simulink model "qless_forgetting_factor_16x16"  (R2021a)
settings: Solver=FixedStepDiscrete  StartTime=0.0  StopTime=stoptime*inf  RelTol=1e-3
InitFcn:
  | qless_init_16chan_fi
undefined symbols (not defined in the file): fc, numArrayElements, physconst, srcAngles, sv, Ts
libraries: hdlsllib x137, commfilt2 x4, commrfcorlib x3, commsync2 x3, commrflib2 x2, commrandsrc3 x2, phasedtxrxlib x2, commdigbbndcpm2 x1, simulink x1, embreciprocals x1, commdigbbndpm3 x1
(part 4 of 22)

== system qless_forgetting_factor_16x16/MVDR_QLess_HDL/Complex Partial-Systolic Matrix Solve Using Q-less QR Decomposition with Forgetting Factor Manually Tiled n=16/Complex Partial-Systolic Q-less QR with Forgetting Factor/Complex Partial-Systolic Q-less QR with Forgetting Factor Manually tiled/Complex Partial-Systolic Q-less QR Decomposition with Forgetting Factor Section Constant pivot9 ==
  "A(i, :)^T" : Inport
  validIn : Inport  Port=2
  restart : Inport  Port=3
  Complex Partial-Systolic Q-less QR Row Rotations : Subsystem  mask(QR Complex Row Rotations){n=n, pivot=pivot}
      mask prompts: n "fixed:emblib:ColumnsInA"
      mask help: fixed:emblib:ComplexRowRotationsFullDescription
      mask DialogControl n Prompt: Number of columns in matrix A
  Data Type Conversion{,2..6} (6 alike) : DataTypeConversion  OutDataTypeStr=boolean
  Forgetting Factor : Gain  Gain=forgettingFactor  OutDataTypeStr=Inherit: Same as input
  Partial-Systolic Q-less QR with Forgetting Factor Memory Controller : Subsystem  TreatAsAtomicUnit=on  mask(Burst Q-less QR QR Memory Controller){n=n}
      mask prompts: n "fixed:emblib:ColumnsInA"
      mask help: fixed:emblib:MemoryControllerDescription
      mask DialogControl n Prompt: Number of columns in matrix A
  Same Datatype : Subsystem  TreatAsAtomicUnit=on
  Terminator : Terminator
  "R(i, :)^T" : Outport  VectorParamsAs1DForOutWhenUnconnected=off
  validR : Outport  Port=2  VectorParamsAs1DForOutWhenUnconnected=off
  yOut : Outport  Port=3  VectorParamsAs1DForOutWhenUnconnected=off
  validY : Outport  Port=4  VectorParamsAs1DForOutWhenUnconnected=off
  ready : Outport  Port=5  VectorParamsAs1DForOutWhenUnconnected=off
  wires:
  "A(i, :)^T"/1 -> Same Datatype/2(Reference), Partial-Systolic Q-less QR with Forgetting Factor Memory Controller/2(aIn)
  restart/1 -> Data Type Conversion2/1
  Complex Partial-Systolic Q-less QR Row Rotations/3(validOut) -> Data Type Conversion3/1
  Partial-Systolic Q-less QR with Forgetting Factor Memory Controller/4(validOut) -> Data Type Conversion5/1
  validIn/1 -> Data Type Conversion/1
  Partial-Systolic Q-less QR with Forgetting Factor Memory Controller/2(yOut) -> Complex Partial-Systolic Q-less QR Row Rotations/2(y)
  Same Datatype/1(DataOut) -> Partial-Systolic Q-less QR with Forgetting Factor Memory Controller/1(xIn)
  Partial-Systolic Q-less QR with Forgetting Factor Memory Controller/5(ready) -> Data Type Conversion6/1
  Complex Partial-Systolic Q-less QR Row Rotations/2(yOut) -> yOut/1
  Complex Partial-Systolic Q-less QR Row Rotations/4(ready) -> Terminator/1
  Partial-Systolic Q-less QR with Forgetting Factor Memory Controller/3(process) -> Data Type Conversion4/1
  Complex Partial-Systolic Q-less QR Row Rotations/1(xOut) -> Forgetting Factor/1
  Partial-Systolic Q-less QR with Forgetting Factor Memory Controller/1(xOut) -> Complex Partial-Systolic Q-less QR Row Rotations/1(x), "R(i, :)^T"/1
  Forgetting Factor/1 -> Same Datatype/1(Data)
  Data Type Conversion/1 -> Partial-Systolic Q-less QR with Forgetting Factor Memory Controller/3(validIn)
  Data Type Conversion2/1 -> Complex Partial-Systolic Q-less QR Row Rotations/4(restart), Partial-Systolic Q-less QR with Forgetting Factor Memory Controller/5(restart)
  Data Type Conversion3/1 -> Partial-Systolic Q-less QR with Forgetting Factor Memory Controller/4(validElim), validY/1
  Data Type Conversion5/1 -> validR/1
  Data Type Conversion6/1 -> ready/1
  Data Type Conversion4/1 -> Complex Partial-Systolic Q-less QR Row Rotations/3(validIn)

== system qless_forgetting_factor_16x16/MVDR_QLess_HDL/Complex Partial-Systolic Matrix Solve Using Q-less QR Decomposition with Forgetting Factor Manually Tiled n=16/Complex Partial-Systolic Q-less QR with Forgetting Factor/Complex Partial-Systolic Q-less QR with Forgetting Factor Manually tiled/Lengthen ==
  u : Inport
  Lengthen : MATLAB Function  TreatAsAtomicUnit=on
  y : Outport
  wires:
  Lengthen/1(y) -> y/1
  u/1 -> Lengthen/1(u)

== system qless_forgetting_factor_16x16/MVDR_QLess_HDL/Complex Partial-Systolic Matrix Solve Using Q-less QR Decomposition with Forgetting Factor Manually Tiled n=16/Complex Partial-Systolic Q-less QR with Forgetting Factor/Complex Partial-Systolic Q-less QR with Forgetting Factor Manually tiled/Lengthen1 ==
  u : Inport
  Lengthen : MATLAB Function  TreatAsAtomicUnit=on
  y : Outport
  wires:
  Lengthen/1(y) -> y/1
  u/1 -> Lengthen/1(u)

== system qless_forgetting_factor_16x16/MVDR_QLess_HDL/Complex Partial-Systolic Matrix Solve Using Q-less QR Decomposition with Forgetting Factor Manually Tiled n=16/Complex Partial-Systolic Q-less QR with Forgetting Factor/Complex Partial-Systolic Q-less QR with Forgetting Factor Manually tiled/Lengthen10 ==
  u : Inport
  Lengthen : MATLAB Function  TreatAsAtomicUnit=on
  y : Outport
  wires:
  Lengthen/1(y) -> y/1
  u/1 -> Lengthen/1(u)

== system qless_forgetting_factor_16x16/MVDR_QLess_HDL/Complex Partial-Systolic Matrix Solve Using Q-less QR Decomposition with Forgetting Factor Manually Tiled n=16/Complex Partial-Systolic Q-less QR with Forgetting Factor/Complex Partial-Systolic Q-less QR with Forgetting Factor Manually tiled/Lengthen11 ==
  u : Inport
  Lengthen : MATLAB Function  TreatAsAtomicUnit=on
  y : Outport
  wires:
  Lengthen/1(y) -> y/1
  u/1 -> Lengthen/1(u)

== system qless_forgetting_factor_16x16/MVDR_QLess_HDL/Complex Partial-Systolic Matrix Solve Using Q-less QR Decomposition with Forgetting Factor Manually Tiled n=16/Complex Partial-Systolic Q-less QR with Forgetting Factor/Complex Partial-Systolic Q-less QR with Forgetting Factor Manually tiled/Lengthen12 ==
  u : Inport
  Lengthen : MATLAB Function  TreatAsAtomicUnit=on
  y : Outport
  wires:
  Lengthen/1(y) -> y/1
  u/1 -> Lengthen/1(u)

== system qless_forgetting_factor_16x16/MVDR_QLess_HDL/Complex Partial-Systolic Matrix Solve Using Q-less QR Decomposition with Forgetting Factor Manually Tiled n=16/Complex Partial-Systolic Q-less QR with Forgetting Factor/Complex Partial-Systolic Q-less QR with Forgetting Factor Manually tiled/Lengthen13 ==
  u : Inport
  Lengthen : MATLAB Function  TreatAsAtomicUnit=on
  y : Outport
  wires:
  Lengthen/1(y) -> y/1
  u/1 -> Lengthen/1(u)

== system qless_forgetting_factor_16x16/MVDR_QLess_HDL/Complex Partial-Systolic Matrix Solve Using Q-less QR Decomposition with Forgetting Factor Manually Tiled n=16/Complex Partial-Systolic Q-less QR with Forgetting Factor/Complex Partial-Systolic Q-less QR with Forgetting Factor Manually tiled/Lengthen14 ==
  u : Inport
  Lengthen : MATLAB Function  TreatAsAtomicUnit=on
  y : Outport
  wires:
  Lengthen/1(y) -> y/1
  u/1 -> Lengthen/1(u)

== system qless_forgetting_factor_16x16/MVDR_QLess_HDL/Complex Partial-Systolic Matrix Solve Using Q-less QR Decomposition with Forgetting Factor Manually Tiled n=16/Complex Partial-Systolic Q-less QR with Forgetting Factor/Complex Partial-Systolic Q-less QR with Forgetting Factor Manually tiled/Lengthen2 ==
  u : Inport
  Lengthen : MATLAB Function  TreatAsAtomicUnit=on
  y : Outport
  wires:
  Lengthen/1(y) -> y/1
  u/1 -> Lengthen/1(u)

== system qless_forgetting_factor_16x16/MVDR_QLess_HDL/Complex Partial-Systolic Matrix Solve Using Q-less QR Decomposition with Forgetting Factor Manually Tiled n=16/Complex Partial-Systolic Q-less QR with Forgetting Factor/Complex Partial-Systolic Q-less QR with Forgetting Factor Manually tiled/Lengthen3 ==
  u : Inport
  Lengthen : MATLAB Function  TreatAsAtomicUnit=on
  y : Outport
  wires:
  Lengthen/1(y) -> y/1
  u/1 -> Lengthen/1(u)

== system qless_forgetting_factor_16x16/MVDR_QLess_HDL/Complex Partial-Systolic Matrix Solve Using Q-less QR Decomposition with Forgetting Factor Manually Tiled n=16/Complex Partial-Systolic Q-less QR with Forgetting Factor/Complex Partial-Systolic Q-less QR with Forgetting Factor Manually tiled/Lengthen4 ==
  u : Inport
  Lengthen : MATLAB Function  TreatAsAtomicUnit=on
  y : Outport
  wires:
  Lengthen/1(y) -> y/1
  u/1 -> Lengthen/1(u)

== system qless_forgetting_factor_16x16/MVDR_QLess_HDL/Complex Partial-Systolic Matrix Solve Using Q-less QR Decomposition with Forgetting Factor Manually Tiled n=16/Complex Partial-Systolic Q-less QR with Forgetting Factor/Complex Partial-Systolic Q-less QR with Forgetting Factor Manually tiled/Lengthen5 ==
  u : Inport
  Lengthen : MATLAB Function  TreatAsAtomicUnit=on
  y : Outport
  wires:
  Lengthen/1(y) -> y/1
  u/1 -> Lengthen/1(u)

== system qless_forgetting_factor_16x16/MVDR_QLess_HDL/Complex Partial-Systolic Matrix Solve Using Q-less QR Decomposition with Forgetting Factor Manually Tiled n=16/Complex Partial-Systolic Q-less QR with Forgetting Factor/Complex Partial-Systolic Q-less QR with Forgetting Factor Manually tiled/Lengthen6 ==
  u : Inport
  Lengthen : MATLAB Function  TreatAsAtomicUnit=on
  y : Outport
  wires:
  Lengthen/1(y) -> y/1
  u/1 -> Lengthen/1(u)

== system qless_forgetting_factor_16x16/MVDR_QLess_HDL/Complex Partial-Systolic Matrix Solve Using Q-less QR Decomposition with Forgetting Factor Manually Tiled n=16/Complex Partial-Systolic Q-less QR with Forgetting Factor/Complex Partial-Systolic Q-less QR with Forgetting Factor Manually tiled/Lengthen7 ==
  u : Inport
  Lengthen : MATLAB Function  TreatAsAtomicUnit=on
  y : Outport
  wires:
  Lengthen/1(y) -> y/1
  u/1 -> Lengthen/1(u)

== system qless_forgetting_factor_16x16/MVDR_QLess_HDL/Complex Partial-Systolic Matrix Solve Using Q-less QR Decomposition with Forgetting Factor Manually Tiled n=16/Complex Partial-Systolic Q-less QR with Forgetting Factor/Complex Partial-Systolic Q-less QR with Forgetting Factor Manually tiled/Lengthen8 ==
  u : Inport
  Lengthen : MATLAB Function  TreatAsAtomicUnit=on
  y : Outport
  wires:
  Lengthen/1(y) -> y/1
  u/1 -> Lengthen/1(u)

== system qless_forgetting_factor_16x16/MVDR_QLess_HDL/Complex Partial-Systolic Matrix Solve Using Q-less QR Decomposition with Forgetting Factor Manually Tiled n=16/Complex Partial-Systolic Q-less QR with Forgetting Factor/Complex Partial-Systolic Q-less QR with Forgetting Factor Manually tiled/Lengthen9 ==
  u : Inport
  Lengthen : MATLAB Function  TreatAsAtomicUnit=on
  y : Outport
  wires:
  Lengthen/1(y) -> y/1
  u/1 -> Lengthen/1(u)

== system qless_forgetting_factor_16x16/MVDR_QLess_HDL/Complex Partial-Systolic Matrix Solve Using Q-less QR Decomposition with Forgetting Factor Manually Tiled n=16/Complex Partial-Systolic Q-less QR with Forgetting Factor/Partial-Systolic Q-less QR with Forgetting Factor Output Memory Manager/Partial-Systolic Q-less QR Output Memory Manager1 ==
  RtransposeIn : Inport
  validIn : Inport  Port=2
  restart : Inport  Port=3
  Delay3 : Delay  DelayLength=1
  Delay5 : Delay  DelayLength=1
  Partial-Systolic Q-less QR Output State Machine : MATLAB Function  TreatAsAtomicUnit=on  mask{m=m, n=n}
      mask prompts: m "fixed:emblib:RowsInA"; n "fixed:emblib:ColumnsInA"
  Save Matrix Row : Subsystem  mask{n=n}
      mask prompts: n "Number of elements in vactor dataIn"
      mask help: The n-by-n input matrix is flattened to an1-by-n^2 row. The row selector is a 1-by-n vector of logical values with a true element corresponding to a row of the matrix to save. There is one cycle delay between input and output.
      mask Display: disp('Save matrix row')
  RtransposeOut : Outport
  validOut : Outport  Port=2
  wires:
  Save Matrix Row/1(matrixOut) -> RtransposeOut/1
  Partial-Systolic Q-less QR Output State Machine/2(validOut) -> Delay3/1
  restart/1 -> Partial-Systolic Q-less QR Output State Machine/2(restart)
  Partial-Systolic Q-less QR Output State Machine/1(writeEnable) -> Save Matrix Row/2(rowSelector)
  Delay5/1 -> Save Matrix Row/1(matrixIn)
  Delay3/1 -> validOut/1
  RtransposeIn/1 -> Delay5/1
  validIn/1 -> Partial-Systolic Q-less QR Output State Machine/1(validIn)

== system qless_forgetting_factor_16x16/MVDR_QLess_HDL/Complex Partial-Systolic Matrix Solve Using Q-less QR Decomposition with Forgetting Factor Manually Tiled n=16/Complex Q-less QR Forward Backward Substitute/Complex Burst Back Substitute with Matrix Output1/Back substitute logic ==
  inverseElement : Inport
  inverseShift : Inport  Port=2
  rIn : Inport  Port=3
  cIn : Inport  Port=4
  validIn : Inport  Port=5
  start : Inport  Port=6
  restart : Inport  Port=7
  Add products : Sum  OutDataTypeStr=Inherit: Same as first input
  Back substitute state machine : MATLAB Function  TreatAsAtomicUnit=on
  Complex-Complex Multiply : Subsystem  TreatAsAtomicUnit=on
  Complex-Real Multiply : Subsystem  TreatAsAtomicUnit=on
  Delay{3..4,8,11} (4 alike) : Delay  DelayLength=1
  Same Datatype : Subsystem  TreatAsAtomicUnit=on
  Same Datatype1 : Subsystem  TreatAsAtomicUnit=on
  Same Datatype2 : Subsystem  TreatAsAtomicUnit=on
  Same Datatype3 : Subsystem  TreatAsAtomicUnit=on
  Subtract sumOfProducts from qtbRow : Sum  Inputs=+-  OutDataTypeStr=Inherit: Same as first input
  Variable shift : Subsystem  TreatAsAtomicUnit=on
  X : Outport  VectorParamsAs1DForOutWhenUnconnected=off
  validOut : Outport  Port=2  VectorParamsAs1DForOutWhenUnconnected=off
  rowReady : Outport  Port=3  VectorParamsAs1DForOutWhenUnconnected=off
  ready : Outport  Port=4  VectorParamsAs1DForOutWhenUnconnected=off
  wires:
  Back substitute state machine/10(xMatrix) -> X/1
  Delay3/1 -> Same Datatype3/1(Data)
  Same Datatype3/1(DataOut) -> Back substitute state machine/11(finalMultipliedRow)
  Delay4/1 -> Same Datatype2/1(Data)
  Same Datatype2/1(DataOut) -> Back substitute state machine/10(multipliedRow)
  Delay8/1 -> Same Datatype1/1(Data)
  Same Datatype1/1(DataOut) -> Back substitute state machine/9(addedRow)
  Delay11/1 -> Same Datatype/1(Data)
  Same Datatype/1(DataOut) -> Back substitute state machine/8(subtractedRow)
  Back substitute state machine/3(rowToAdd1) -> Add products/1
  Back substitute state machine/4(rowToAdd2) -> Add products/2
  Back substitute state machine/6(rElement) -> Complex-Complex Multiply/2(multiplier)
  Back substitute state machine/5(rowToMultiply) -> Complex-Complex Multiply/1(row)
  inverseElement/1 -> Back substitute state machine/1(inverseElement)
  rIn/1 -> Back substitute state machine/3(rIn)
  cIn/1 -> Same Datatype3/2(Reference), Same Datatype2/2(Reference), Same Datatype1/2(Reference), Same Datatype/2(Reference), Back substitute state machine/4(cIn)
  validIn/1 -> Back substitute state machine/5(validIn)
  start/1 -> Back substitute state machine/6(start)
  restart/1 -> Back substitute state machine/7(restart)
  Back substitute state machine/11(ready) -> ready/1
  Back substitute state machine/12(rowReady) -> rowReady/1
  Back substitute state machine/9(shiftValue) -> Variable shift/2(shiftValue)
  inverseShift/1 -> Back substitute state machine/2(inverseShift)
  Back substitute state machine/13(validOut) -> validOut/1
  Back substitute state machine/8(reciprocal) -> Complex-Real Multiply/2(multiplier)
  Back substitute state machine/7(finalRowToMultiply) -> Complex-Real Multiply/1(row)
  Complex-Real Multiply/1(output) -> Variable shift/1(x)
  Variable shift/1(y) -> Delay3/1
  Complex-Complex Multiply/1(output) -> Delay4/1
  Back substitute state machine/2(rowToSubtract2) -> Subtract sumOfProducts from qtbRow/2
  Back substitute state machine/1(rowToSubtract1) -> Subtract sumOfProducts from qtbRow/1
  Subtract sumOfProducts from qtbRow/1 -> Delay11/1
  Add products/1 -> Delay8/1

== system qless_forgetting_factor_16x16/MVDR_QLess_HDL/Complex Partial-Systolic Matrix Solve Using Q-less QR Decomposition with Forgetting Factor Manually Tiled n=16/Complex Q-less QR Forward Backward Substitute/Complex Burst Back Substitute with Matrix Output1/Reciprocal of the diagonal element ==
  rIn : Inport
  start : Inport  Port=2
  validIn : Inport  Port=3
  Positive Normalized Reciprocal HDL Optimized : Subsystem  mask(Positive Normalized Reciprocal HDL Optimized){}
      mask help: fixed:emblib:PositiveNormalizedReciprocalFullDescription
      mask Help: For internal use only. This feature is intentionally undocumented. Its behavior may change, or it may be removed in a future release.
      mask Display:
      | text(0.5,0.7,'u > 0','texmode','on','HorizontalAlignment','center')
      | text(0.5,0.5,'2^e y = 1/u','texmode','on','HorizontalAlignment','center')
      | text(0.5,0.3,'0.5 < y \leq 1','texmode','on','HorizontalAlignment','center')
  Select diagonal element : MATLAB Function  TreatAsAtomicUnit=on
  inverseElement : Outport  VectorParamsAs1DForOutWhenUnconnected=off
  inverseShift : Outport  Port=2  VectorParamsAs1DForOutWhenUnconnected=off
  validOut : Outport  Port=3  VectorParamsAs1DForOutWhenUnconnected=off
  wires:
  Positive Normalized Reciprocal HDL Optimized/2(e) -> inverseShift/1
  Positive Normalized Reciprocal HDL Optimized/3(validOut) -> validOut/1
  Select diagonal element/1(y) -> Positive Normalized Reciprocal HDL Optimized/1(u)
  rIn/1 -> Select diagonal element/1(rIn)
  Select diagonal element/2(validOut) -> Positive Normalized Reciprocal HDL Optimized/2(validIn)
  start/1 -> Select diagonal element/2(start)
  validIn/1 -> Select diagonal element/3(validIn)
  Positive Normalized Reciprocal HDL Optimized/1(y) -> inverseElement/1

== system qless_forgetting_factor_16x16/MVDR_QLess_HDL/Complex Partial-Systolic Matrix Solve Using Q-less QR Decomposition with Forgetting Factor Manually Tiled n=16/Complex Q-less QR Forward Backward Substitute/Complex Burst Forward Substitute with Matrix Output/Forward substitute logic ==
  inverseElement : Inport
  inverseShift : Inport  Port=2
  rIn : Inport  Port=3
  cIn : Inport  Port=4
  validIn : Inport  Port=5
  start : Inport  Port=6
  restart : Inport  Port=7
  Add products : Sum  OutDataTypeStr=Inherit: Same as first input
  Complex-Complex Multiply1 : Subsystem  TreatAsAtomicUnit=on
  Complex-Real Multiply : Subsystem  TreatAsAtomicUnit=on
  Delay{3..4,8,11} (4 alike) : Delay  DelayLength=1
  Forward substitute state machine : MATLAB Function  TreatAsAtomicUnit=on
  Same Datatype : Subsystem  TreatAsAtomicUnit=on
  Same Datatype1 : Subsystem  TreatAsAtomicUnit=on
  Same Datatype2 : Subsystem  TreatAsAtomicUnit=on
  Same Datatype3 : Subsystem  TreatAsAtomicUnit=on
  Subtract sumOfProducts from qtbRow : Sum  Inputs=+-  OutDataTypeStr=Inherit: Same as first input
  Variable shift : Subsystem  TreatAsAtomicUnit=on
  X : Outport  VectorParamsAs1DForOutWhenUnconnected=off
  validOut : Outport  Port=2  VectorParamsAs1DForOutWhenUnconnected=off
  rowReady : Outport  Port=3  VectorParamsAs1DForOutWhenUnconnected=off
  ready : Outport  Port=4  VectorParamsAs1DForOutWhenUnconnected=off
  wires:
  Forward substitute state machine/10(xMatrix) -> X/1
  Forward substitute state machine/13(validOut) -> validOut/1
  Delay3/1 -> Same Datatype3/1(Data)
  Same Datatype3/1(DataOut) -> Forward substitute state machine/11(finalMultipliedRow)
  Delay4/1 -> Same Datatype2/1(Data)
  Same Datatype2/1(DataOut) -> Forward substitute state machine/10(multipliedRow)
  Delay8/1 -> Same Datatype1/1(Data)
  Same Datatype1/1(DataOut) -> Forward substitute state machine/9(addedRow)
  Delay11/1 -> Same Datatype/1(Data)
  Same Datatype/1(DataOut) -> Forward substitute state machine/8(subtractedRow)
  Forward substitute state machine/3(rowToAdd1) -> Add products/1
  Forward substitute state machine/4(rowToAdd2) -> Add products/2
  Forward substitute state machine/6(rElement) -> Complex-Complex Multiply1/2(multiplier)
  Forward substitute state machine/5(rowToMultiply) -> Complex-Complex Multiply1/1(row)
  inverseElement/1 -> Forward substitute state machine/1(inverseElement)
  rIn/1 -> Forward substitute state machine/3(rIn)
  cIn/1 -> Same Datatype3/2(Reference), Same Datatype2/2(Reference), Same Datatype1/2(Reference), Same Datatype/2(Reference), Forward substitute state machine/4(cIn)
  validIn/1 -> Forward substitute state machine/5(validIn)
  start/1 -> Forward substitute state machine/6(start)
  restart/1 -> Forward substitute state machine/7(restart)
  Forward substitute state machine/11(ready) -> ready/1
  Forward substitute state machine/12(rowReady) -> rowReady/1
  Forward substitute state machine/9(shiftValue) -> Variable shift/2(shiftValue)
  inverseShift/1 -> Forward substitute state machine/2(inverseShift)
  Forward substitute state machine/8(reciprocal) -> Complex-Real Multiply/2(multiplier)
  Forward substitute state machine/7(finalRowToMultiply) -> Complex-Real Multiply/1(row)
  Complex-Real Multiply/1(output) -> Variable shift/1(x)
  Variable shift/1(y) -> Delay3/1
  Complex-Complex Multiply1/1(output) -> Delay4/1
  Forward substitute state machine/2(rowToSubtract2) -> Subtract sumOfProducts from qtbRow/2
  Forward substitute state machine/1(rowToSubtract1) -> Subtract sumOfProducts from qtbRow/1
  Subtract sumOfProducts from qtbRow/1 -> Delay11/1
  Add products/1 -> Delay8/1

== system qless_forgetting_factor_16x16/MVDR_QLess_HDL/Complex Partial-Systolic Matrix Solve Using Q-less QR Decomposition with Forgetting Factor Manually Tiled n=16/Complex Q-less QR Forward Backward Substitute/Complex Burst Forward Substitute with Matrix Output/Reciprocal of the diagonal element ==
  rIn : Inport
  start : Inport  Port=2
  validIn : Inport  Port=3
  Positive Normalized Reciprocal HDL Optimized : Subsystem  mask(Positive Normalized Reciprocal HDL Optimized){}
      mask help: fixed:emblib:PositiveNormalizedReciprocalFullDescription
      mask Help: For internal use only. This feature is intentionally undocumented. Its behavior may change, or it may be removed in a future release.
      mask Display:
      | text(0.5,0.7,'u > 0','texmode','on','HorizontalAlignment','center')
      | text(0.5,0.5,'2^e y = 1/u','texmode','on','HorizontalAlignment','center')
      | text(0.5,0.3,'0.5 < y \leq 1','texmode','on','HorizontalAlignment','center')
  Select diagonal element : MATLAB Function  TreatAsAtomicUnit=on
  inverseElement : Outport  VectorParamsAs1DForOutWhenUnconnected=off
  inverseShift : Outport  Port=2  VectorParamsAs1DForOutWhenUnconnected=off
  validOut : Outport  Port=3  VectorParamsAs1DForOutWhenUnconnected=off
  wires:
  Positive Normalized Reciprocal HDL Optimized/2(e) -> inverseShift/1
  Positive Normalized Reciprocal HDL Optimized/3(validOut) -> validOut/1
  Select diagonal element/1(y) -> Positive Normalized Reciprocal HDL Optimized/1(u)
  rIn/1 -> Select diagonal element/1(rIn)
  Select diagonal element/2(validOut) -> Positive Normalized Reciprocal HDL Optimized/2(validIn)
  start/1 -> Select diagonal element/2(start)
  validIn/1 -> Select diagonal element/3(validIn)
  Positive Normalized Reciprocal HDL Optimized/1(y) -> inverseElement/1

== system qless_forgetting_factor_16x16/MVDR_QLess_HDL/Complex Partial-Systolic Matrix Solve Using Q-less QR Decomposition with Forgetting Factor Manually Tiled n=16/Complex Q-less QR Forward Backward Substitute/Partial-Systolic Matrix Solve Q-less QR B Buffer Manager/Save Matrix B ==
  matrixIn : Inport  Partition=on  PartitionDimension=1  PartitionWidth=n  PartitionOffset=0
  validIn : Inport  Port=2
  restart : Inport  Port=3
  Enabled Delay : MATLAB Function  TreatAsAtomicUnit=on
  For Each : ForEach  DisableCoverage=on
  Reshape : Reshape  OutputDimensionality=Column vector (2-D)
  matrixOut : Outport  ConcatenationDimension=1
  wires:
  restart/1 -> Enabled Delay/3(restart)
  validIn/1 -> Enabled Delay/2(writeEnable)
  matrixIn/1 -> Enabled Delay/1(dataIn)
  Enabled Delay/1(dataOut) -> Reshape/1
  Reshape/1 -> matrixOut/1

== system qless_forgetting_factor_16x16/MVDR_QLess_HDL/Complex Partial-Systolic Matrix Solve Using Q-less QR Decomposition with Forgetting Factor Manually Tiled n=16/Complex Q-less QR Forward Backward Substitute/Partial-Systolic Matrix Solve Q-less QR Forward Substitute Memory Manager/Save Matrix B ==
  matrixIn : Inport  Partition=on  PartitionDimension=1  PartitionWidth=n  PartitionOffset=0
  validIn : Inport  Port=2
  restart : Inport  Port=3
  Enabled Delay : MATLAB Function  TreatAsAtomicUnit=on
  For Each : ForEach  DisableCoverage=on
  Reshape : Reshape  OutputDimensionality=Column vector (2-D)
  matrixOut : Outport  ConcatenationDimension=1
  wires:
  restart/1 -> Enabled Delay/3(restart)
  validIn/1 -> Enabled Delay/2(writeEnable)
  matrixIn/1 -> Enabled Delay/1(dataIn)
  Enabled Delay/1(dataOut) -> Reshape/1
  Reshape/1 -> matrixOut/1

== system qless_forgetting_factor_16x16/MVDR_QLess_HDL/Complex Partial-Systolic Matrix Solve Using Q-less QR Decomposition with Forgetting Factor Manually Tiled n=16/Complex Q-less QR Forward Backward Substitute/Partial-Systolic Matrix Solve Q-less QR Output Manager/Save Matrix ==
  matrixIn : Inport  Partition=on  PartitionDimension=1  PartitionWidth=n  PartitionOffset=0
  validIn : Inport  Port=2
  restart : Inport  Port=3
  Enabled Delay : MATLAB Function  TreatAsAtomicUnit=on
  For Each : ForEach  DisableCoverage=on
  Reshape : Reshape  OutputDimensionality=Column vector (2-D)
  matrixOut : Outport  ConcatenationDimension=1
  wires:
  restart/1 -> Enabled Delay/3(restart)
  validIn/1 -> Enabled Delay/2(writeEnable)
  matrixIn/1 -> Enabled Delay/1(dataIn)
  Enabled Delay/1(dataOut) -> Reshape/1
  Reshape/1 -> matrixOut/1

== system qless_forgetting_factor_16x16/MVDR_QLess_HDL/Normalize Response/MVDR Weight Update/Inner Product/Element-wise complex product ==
  u : Inport  Partition=on  PartitionDimension=1  PartitionWidth=1  PartitionOffset=0
  v : Inport  Port=2  Partition=on  PartitionDimension=1  PartitionWidth=1  PartitionOffset=0
  For Each : ForEach  DisableCoverage=on
  HDL Complex Multiply : Subsystem  mask(HDL Complex Multiplier (3 Multiply, 5 Add)){D1=2, D2=1, D3=1, D4=1, D5=1}
      mask help:
      | Xilinx devices:
      | - Set D1 = 1 or 2 to trade off speed & FF resources
      | - Set D2-D5 = 1 to fully leverage DSP48 pipelines
      | - Use sync reset
      |
      | Intel FPGAs:
      | - Set D1 = 1 or 2 depending on device family
      | - Set D5 = 1; D2, D3, D4 = 0
      | - Use async reset
      mask init:
      | delay = D1+D2+D3+D4+D5;
      mask Display:
      | fprintf('Delay=%d',delay);
      | port_label('input',1,'z1');
      | port_label('input',2,'z2');
  y : Outport  ConcatenationDimension=1
  wires:
  v/1 -> HDL Complex Multiply/2(In2)
  HDL Complex Multiply/1(Out1) -> y/1
  u/1 -> HDL Complex Multiply/1(In1)

== system qless_forgetting_factor_16x16/MVDR_QLess_HDL/Normalize Response/MVDR Weight Update/Inner Product/Tree Sum with Distributed Pipelining ==
  In1 : Inport
  Delay3 : Delay  DelayLength=ceil(log2(numArrayElements))
  Tree Sum of Elements : Sum  Inputs=+
  Out1 : Outport
  wires:
  Delay3/1 -> Out1/1
  In1/1 -> Tree Sum of Elements/1
  Tree Sum of Elements/1 -> Delay3/1

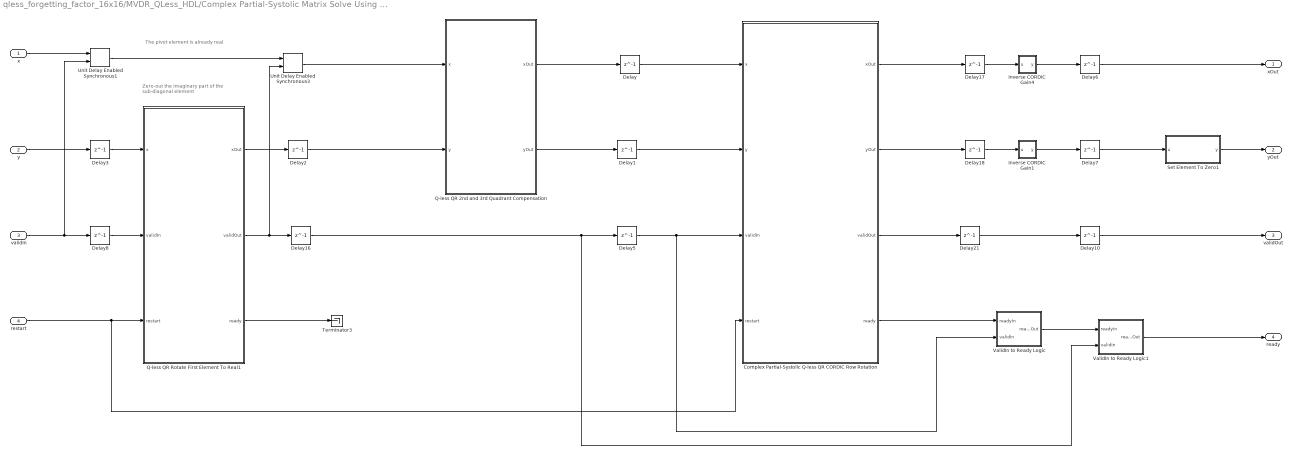
== system qless_forgetting_factor_16x16/MVDR_QLess_HDL/Complex Partial-Systolic Matrix Solve Using Q-less QR Decomposition with Forgetting Factor Manually Tiled n=16/Complex Partial-Systolic Q-less QR with Forgetting Factor/Complex Partial-Systolic Q-less QR with Forgetting Factor Manually tiled/Complex Partial-Systolic Q-less QR Decomposition with Forgetting Factor Section Constant pivot1/Complex Partial-Systolic Q-less QR Row Rotations ==
  note: The pivot element is already real
  note: Zero-out the imaginary part
      | of the sub-diagonal element
  x : Inport
  y : Inport  Port=2
  validIn : Inport  Port=3
  restart : Inport  Port=4
  Complex Partial-Systolic Q-less QR CORDIC Row Rotation : Subsystem  TreatAsAtomicUnit=on  mask(Real Indexed CORDIC Row Rotation){n=n, pivot=pivot}
      mask prompts: n "fixed:emblib:ColumnsInA"
      mask help: fixed:emblib:RealIdxCORDIC
      mask DialogControl n Prompt: Number of columns in matrix A
  Delay{,1..3,5..8,10,16..18,21} (13 alike) : Delay  DelayLength=1
  Inverse CORDIC Gain1 : Subsystem  mask(Inverse CORDIC Gain){}
      mask help: fixed:emblib:InverseCORDICGainDescription
      mask Display: disp('1/An')
  Inverse CORDIC Gain4 : Subsystem  mask(Inverse CORDIC Gain){}
      mask help: fixed:emblib:InverseCORDICGainDescription
      mask Display: disp('1/An')
  Q-less QR 2nd and 3rd Quadrant Compensation : MATLAB Function  TreatAsAtomicUnit=on
  Q-less QR Rotate First Element To Real1 : Subsystem  TreatAsAtomicUnit=on  mask(Rotate First Element To Real){n=n, pivot=pivot}
      mask prompts: n "fixed:emblib:ColumnsInA"
      mask help: fixed:emblib:RotateFirstElementToRealDescription
      mask DialogControl n Prompt: Number of columns in matrix A
  Set Element To Zero1 : Subsystem  mask(Set Element To Zero){n=n, pivot=pivot}
      mask prompts: n "fixed:emblib:ColumnsInA"
      mask help: fixed:emblib:SetElementToZeroDescription
      mask DialogControl n Prompt: Number of columns in matrix A
  Terminator3 : Terminator
  Unit Delay Enabled Synchronous1 : hdlsllib/Discrete/Unit Delay Enabled Synchronous  InitialCondition=0.0  SampleTime=-1
      settings: SourceProductBaseCode=SL
  Unit Delay Enabled Synchronous3 : hdlsllib/Discrete/Unit Delay Enabled Synchronous  InitialCondition=0.0  SampleTime=-1
      settings: SourceProductBaseCode=SL
  ValidIn to Ready Logic : Subsystem
  ValidIn to Ready Logic1 : Subsystem
  xOut : Outport  VectorParamsAs1DForOutWhenUnconnected=off
  yOut : Outport  Port=2  VectorParamsAs1DForOutWhenUnconnected=off
  validOut : Outport  Port=3  VectorParamsAs1DForOutWhenUnconnected=off
  ready : Outport  Port=4  VectorParamsAs1DForOutWhenUnconnected=off
  wires:
  Delay6/1 -> xOut/1
  Complex Partial-Systolic Q-less QR CORDIC Row Rotation/1(xOut) -> Delay17/1
  Q-less QR 2nd and 3rd Quadrant Compensation/1(xOut) -> Delay/1
  Q-less QR 2nd and 3rd Quadrant Compensation/2(yOut) -> Delay1/1
  Delay/1 -> Complex Partial-Systolic Q-less QR CORDIC Row Rotation/1(x)
  Q-less QR Rotate First Element To Real1/2(validOut) -> Unit Delay Enabled Synchronous3/2, Delay16/1
  Q-less QR Rotate First Element To Real1/1(xOut) -> Delay2/1
  Delay1/1 -> Complex Partial-Systolic Q-less QR CORDIC Row Rotation/2(y)
  restart/1 -> Q-less QR Rotate First Element To Real1/3(restart), Complex Partial-Systolic Q-less QR CORDIC Row Rotation/4(restart)
  Delay5/1 -> ValidIn to Ready Logic/2(validIn), Complex Partial-Systolic Q-less QR CORDIC Row Rotation/3(validIn)
  Complex Partial-Systolic Q-less QR CORDIC Row Rotation/4(ready) -> ValidIn to Ready Logic/1(readyIn)
  Complex Partial-Systolic Q-less QR CORDIC Row Rotation/3(validOut) -> Delay21/1
  Complex Partial-Systolic Q-less QR CORDIC Row Rotation/2(yOut) -> Delay18/1
  y/1 -> Delay3/1
  Delay10/1 -> validOut/1
  ValidIn to Ready Logic/1(readyOut) -> ValidIn to Ready Logic1/1(readyIn)
  Delay7/1 -> Set Element To Zero1/1(u)
  Q-less QR Rotate First Element To Real1/3(ready) -> Terminator3/1
  ValidIn to Ready Logic1/1(readyOut) -> ready/1
  Delay21/1 -> Delay10/1
  Delay18/1 -> Inverse CORDIC Gain1/1(u)
  Delay17/1 -> Inverse CORDIC Gain4/1(u)
  Inverse CORDIC Gain4/1(y) -> Delay6/1
  Inverse CORDIC Gain1/1(y) -> Delay7/1
  validIn/1 -> Unit Delay Enabled Synchronous1/2, Delay8/1
  Delay16/1 -> ValidIn to Ready Logic1/2(validIn), Delay5/1
  Delay2/1 -> Q-less QR 2nd and 3rd Quadrant Compensation/2(y)
  Unit Delay Enabled Synchronous3/1 -> Q-less QR 2nd and 3rd Quadrant Compensation/1(x)
  Unit Delay Enabled Synchronous1/1 -> Unit Delay Enabled Synchronous3/1
  x/1 -> Unit Delay Enabled Synchronous1/1
  Delay3/1 -> Q-less QR Rotate First Element To Real1/1(x)
  Delay8/1 -> Q-less QR Rotate First Element To Real1/2(validIn)
  Set Element To Zero1/1(y) -> yOut/1

== system qless_forgetting_factor_16x16/MVDR_QLess_HDL/Complex Partial-Systolic Matrix Solve Using Q-less QR Decomposition with Forgetting Factor Manually Tiled n=16/Complex Partial-Systolic Q-less QR with Forgetting Factor/Complex Partial-Systolic Q-less QR with Forgetting Factor Manually tiled/Complex Partial-Systolic Q-less QR Decomposition with Forgetting Factor Section Constant pivot1/Partial-Systolic Q-less QR with Forgetting Factor Memory Controller ==
  xIn : Inport
  aIn : Inport  Port=2
  validIn : Inport  Port=3
  validElim : Inport  Port=4
  restart : Inport  Port=5
  Delay{,2..4,6} (5 alike) : Delay  DelayLength=1
  MATLAB Function : MATLAB Function  TreatAsAtomicUnit=on
  xOut : Outport  VectorParamsAs1DForOutWhenUnconnected=off
  yOut : Outport  Port=2  VectorParamsAs1DForOutWhenUnconnected=off
  process : Outport  Port=3  VectorParamsAs1DForOutWhenUnconnected=off
  validOut : Outport  Port=4  VectorParamsAs1DForOutWhenUnconnected=off
  ready : Outport  Port=5  VectorParamsAs1DForOutWhenUnconnected=off
  wires:
  Delay/1 -> MATLAB Function/1(xIn)
  Delay2/1 -> MATLAB Function/2(aIn)
  Delay3/1 -> MATLAB Function/3(validIn)
  Delay4/1 -> MATLAB Function/4(validRowRotationInput)
  Delay6/1 -> MATLAB Function/5(restart)
  xIn/1 -> Delay/1  "A"
  aIn/1 -> Delay2/1
  validIn/1 -> Delay3/1  "validIn"
  validElim/1 -> Delay4/1  "validElim"
  restart/1 -> Delay6/1  "validElim"
  MATLAB Function/1(xOut) -> xOut/1
  MATLAB Function/2(yOut) -> yOut/1
  MATLAB Function/3(processRowRotations) -> process/1
  MATLAB Function/4(validOut) -> validOut/1
  MATLAB Function/5(ready) -> ready/1

== system qless_forgetting_factor_16x16/MVDR_QLess_HDL/Complex Partial-Systolic Matrix Solve Using Q-less QR Decomposition with Forgetting Factor Manually Tiled n=16/Complex Partial-Systolic Q-less QR with Forgetting Factor/Complex Partial-Systolic Q-less QR with Forgetting Factor Manually tiled/Complex Partial-Systolic Q-less QR Decomposition with Forgetting Factor Section Constant pivot1/Same Datatype ==
  Data : Inport
  Reference : Inport  Port=2
  Data Type Duplicate : DataTypeDuplicate
  DataOut : Outport  VectorParamsAs1DForOutWhenUnconnected=off
  wires:
  Reference/1 -> Data Type Duplicate/2
  Data/1 -> DataOut/1, Data Type Duplicate/1

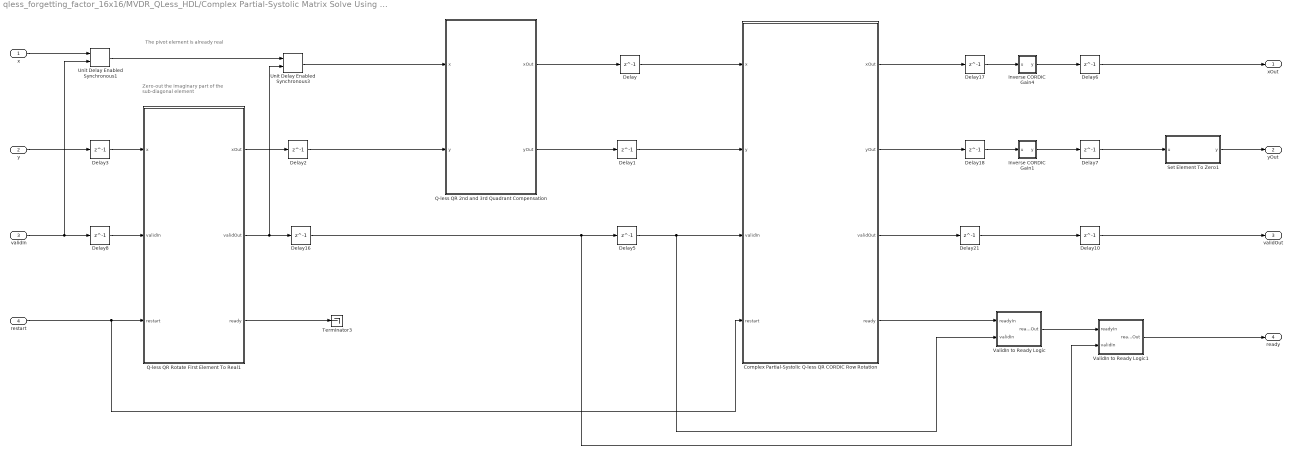
== system qless_forgetting_factor_16x16/MVDR_QLess_HDL/Complex Partial-Systolic Matrix Solve Using Q-less QR Decomposition with Forgetting Factor Manually Tiled n=16/Complex Partial-Systolic Q-less QR with Forgetting Factor/Complex Partial-Systolic Q-less QR with Forgetting Factor Manually tiled/Complex Partial-Systolic Q-less QR Decomposition with Forgetting Factor Section Constant pivot10/Complex Partial-Systolic Q-less QR Row Rotations ==
  note: The pivot element is already real
  note: Zero-out the imaginary part
      | of the sub-diagonal element
  x : Inport
  y : Inport  Port=2
  validIn : Inport  Port=3
  restart : Inport  Port=4
  Complex Partial-Systolic Q-less QR CORDIC Row Rotation : Subsystem  TreatAsAtomicUnit=on  mask(Real Indexed CORDIC Row Rotation){n=n, pivot=pivot}
      mask prompts: n "fixed:emblib:ColumnsInA"
      mask help: fixed:emblib:RealIdxCORDIC
      mask DialogControl n Prompt: Number of columns in matrix A
  Delay{,1..3,5..8,10,16..18,21} (13 alike) : Delay  DelayLength=1
  Inverse CORDIC Gain1 : Subsystem  mask(Inverse CORDIC Gain){}
      mask help: fixed:emblib:InverseCORDICGainDescription
      mask Display: disp('1/An')
  Inverse CORDIC Gain4 : Subsystem  mask(Inverse CORDIC Gain){}
      mask help: fixed:emblib:InverseCORDICGainDescription
      mask Display: disp('1/An')
  Q-less QR 2nd and 3rd Quadrant Compensation : MATLAB Function  TreatAsAtomicUnit=on
  Q-less QR Rotate First Element To Real1 : Subsystem  TreatAsAtomicUnit=on  mask(Rotate First Element To Real){n=n, pivot=pivot}
      mask prompts: n "fixed:emblib:ColumnsInA"
      mask help: fixed:emblib:RotateFirstElementToRealDescription
      mask DialogControl n Prompt: Number of columns in matrix A
  Set Element To Zero1 : Subsystem  mask(Set Element To Zero){n=n, pivot=pivot}
      mask prompts: n "fixed:emblib:ColumnsInA"
      mask help: fixed:emblib:SetElementToZeroDescription
      mask DialogControl n Prompt: Number of columns in matrix A
  Terminator3 : Terminator
  Unit Delay Enabled Synchronous1 : hdlsllib/Discrete/Unit Delay Enabled Synchronous  InitialCondition=0.0  SampleTime=-1
      settings: SourceProductBaseCode=SL
  Unit Delay Enabled Synchronous3 : hdlsllib/Discrete/Unit Delay Enabled Synchronous  InitialCondition=0.0  SampleTime=-1
      settings: SourceProductBaseCode=SL
  ValidIn to Ready Logic : Subsystem
  ValidIn to Ready Logic1 : Subsystem
  xOut : Outport  VectorParamsAs1DForOutWhenUnconnected=off
  yOut : Outport  Port=2  VectorParamsAs1DForOutWhenUnconnected=off
  validOut : Outport  Port=3  VectorParamsAs1DForOutWhenUnconnected=off
  ready : Outport  Port=4  VectorParamsAs1DForOutWhenUnconnected=off
  wires:
  Delay6/1 -> xOut/1
  Complex Partial-Systolic Q-less QR CORDIC Row Rotation/1(xOut) -> Delay17/1
  Q-less QR 2nd and 3rd Quadrant Compensation/1(xOut) -> Delay/1
  Q-less QR 2nd and 3rd Quadrant Compensation/2(yOut) -> Delay1/1
  Delay/1 -> Complex Partial-Systolic Q-less QR CORDIC Row Rotation/1(x)
  Q-less QR Rotate First Element To Real1/2(validOut) -> Unit Delay Enabled Synchronous3/2, Delay16/1
  Q-less QR Rotate First Element To Real1/1(xOut) -> Delay2/1
  Delay1/1 -> Complex Partial-Systolic Q-less QR CORDIC Row Rotation/2(y)
  restart/1 -> Q-less QR Rotate First Element To Real1/3(restart), Complex Partial-Systolic Q-less QR CORDIC Row Rotation/4(restart)
  Delay5/1 -> ValidIn to Ready Logic/2(validIn), Complex Partial-Systolic Q-less QR CORDIC Row Rotation/3(validIn)
  Complex Partial-Systolic Q-less QR CORDIC Row Rotation/4(ready) -> ValidIn to Ready Logic/1(readyIn)
  Complex Partial-Systolic Q-less QR CORDIC Row Rotation/3(validOut) -> Delay21/1
  Complex Partial-Systolic Q-less QR CORDIC Row Rotation/2(yOut) -> Delay18/1
  y/1 -> Delay3/1
  Delay10/1 -> validOut/1
  ValidIn to Ready Logic/1(readyOut) -> ValidIn to Ready Logic1/1(readyIn)
  Delay7/1 -> Set Element To Zero1/1(u)
  Q-less QR Rotate First Element To Real1/3(ready) -> Terminator3/1
  ValidIn to Ready Logic1/1(readyOut) -> ready/1
  Delay21/1 -> Delay10/1
  Delay18/1 -> Inverse CORDIC Gain1/1(u)
  Delay17/1 -> Inverse CORDIC Gain4/1(u)
  Inverse CORDIC Gain4/1(y) -> Delay6/1
  Inverse CORDIC Gain1/1(y) -> Delay7/1
  validIn/1 -> Unit Delay Enabled Synchronous1/2, Delay8/1
  Delay16/1 -> ValidIn to Ready Logic1/2(validIn), Delay5/1
  Delay2/1 -> Q-less QR 2nd and 3rd Quadrant Compensation/2(y)
  Unit Delay Enabled Synchronous3/1 -> Q-less QR 2nd and 3rd Quadrant Compensation/1(x)
  Unit Delay Enabled Synchronous1/1 -> Unit Delay Enabled Synchronous3/1
  x/1 -> Unit Delay Enabled Synchronous1/1
  Delay3/1 -> Q-less QR Rotate First Element To Real1/1(x)
  Delay8/1 -> Q-less QR Rotate First Element To Real1/2(validIn)
  Set Element To Zero1/1(y) -> yOut/1

== system qless_forgetting_factor_16x16/MVDR_QLess_HDL/Complex Partial-Systolic Matrix Solve Using Q-less QR Decomposition with Forgetting Factor Manually Tiled n=16/Complex Partial-Systolic Q-less QR with Forgetting Factor/Complex Partial-Systolic Q-less QR with Forgetting Factor Manually tiled/Complex Partial-Systolic Q-less QR Decomposition with Forgetting Factor Section Constant pivot10/Partial-Systolic Q-less QR with Forgetting Factor Memory Controller ==
  xIn : Inport
  aIn : Inport  Port=2
  validIn : Inport  Port=3
  validElim : Inport  Port=4
  restart : Inport  Port=5
  Delay{,2..4,6} (5 alike) : Delay  DelayLength=1
  MATLAB Function : MATLAB Function  TreatAsAtomicUnit=on
  xOut : Outport  VectorParamsAs1DForOutWhenUnconnected=off
  yOut : Outport  Port=2  VectorParamsAs1DForOutWhenUnconnected=off
  process : Outport  Port=3  VectorParamsAs1DForOutWhenUnconnected=off
  validOut : Outport  Port=4  VectorParamsAs1DForOutWhenUnconnected=off
  ready : Outport  Port=5  VectorParamsAs1DForOutWhenUnconnected=off
  wires:
  Delay/1 -> MATLAB Function/1(xIn)
  Delay2/1 -> MATLAB Function/2(aIn)
  Delay3/1 -> MATLAB Function/3(validIn)
  Delay4/1 -> MATLAB Function/4(validRowRotationInput)
  Delay6/1 -> MATLAB Function/5(restart)
  xIn/1 -> Delay/1  "A"
  aIn/1 -> Delay2/1
  validIn/1 -> Delay3/1  "validIn"
  validElim/1 -> Delay4/1  "validElim"
  restart/1 -> Delay6/1  "validElim"
  MATLAB Function/1(xOut) -> xOut/1
  MATLAB Function/2(yOut) -> yOut/1
  MATLAB Function/3(processRowRotations) -> process/1
  MATLAB Function/4(validOut) -> validOut/1
  MATLAB Function/5(ready) -> ready/1

== system qless_forgetting_factor_16x16/MVDR_QLess_HDL/Complex Partial-Systolic Matrix Solve Using Q-less QR Decomposition with Forgetting Factor Manually Tiled n=16/Complex Partial-Systolic Q-less QR with Forgetting Factor/Complex Partial-Systolic Q-less QR with Forgetting Factor Manually tiled/Complex Partial-Systolic Q-less QR Decomposition with Forgetting Factor Section Constant pivot10/Same Datatype ==
  Data : Inport
  Reference : Inport  Port=2
  Data Type Duplicate : DataTypeDuplicate
  DataOut : Outport  VectorParamsAs1DForOutWhenUnconnected=off
  wires:
  Reference/1 -> Data Type Duplicate/2
  Data/1 -> DataOut/1, Data Type Duplicate/1

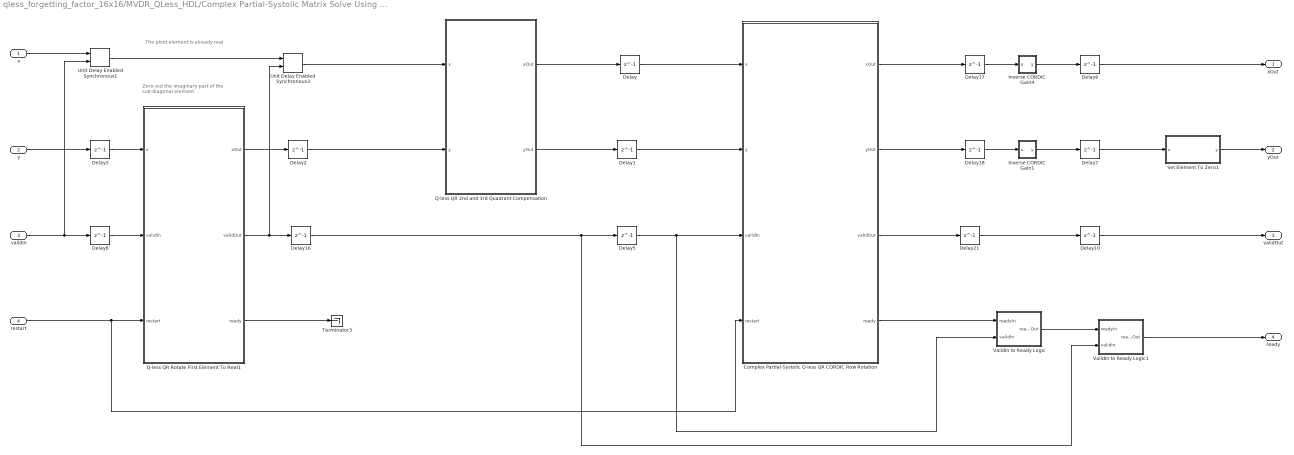
== system qless_forgetting_factor_16x16/MVDR_QLess_HDL/Complex Partial-Systolic Matrix Solve Using Q-less QR Decomposition with Forgetting Factor Manually Tiled n=16/Complex Partial-Systolic Q-less QR with Forgetting Factor/Complex Partial-Systolic Q-less QR with Forgetting Factor Manually tiled/Complex Partial-Systolic Q-less QR Decomposition with Forgetting Factor Section Constant pivot11/Complex Partial-Systolic Q-less QR Row Rotations ==
  note: The pivot element is already real
  note: Zero-out the imaginary part
      | of the sub-diagonal element
  x : Inport
  y : Inport  Port=2
  validIn : Inport  Port=3
  restart : Inport  Port=4
  Complex Partial-Systolic Q-less QR CORDIC Row Rotation : Subsystem  TreatAsAtomicUnit=on  mask(Real Indexed CORDIC Row Rotation){n=n, pivot=pivot}
      mask prompts: n "fixed:emblib:ColumnsInA"
      mask help: fixed:emblib:RealIdxCORDIC
      mask DialogControl n Prompt: Number of columns in matrix A
  Delay{,1..3,5..8,10,16..18,21} (13 alike) : Delay  DelayLength=1
  Inverse CORDIC Gain1 : Subsystem  mask(Inverse CORDIC Gain){}
      mask help: fixed:emblib:InverseCORDICGainDescription
      mask Display: disp('1/An')
  Inverse CORDIC Gain4 : Subsystem  mask(Inverse CORDIC Gain){}
      mask help: fixed:emblib:InverseCORDICGainDescription
      mask Display: disp('1/An')
  Q-less QR 2nd and 3rd Quadrant Compensation : MATLAB Function  TreatAsAtomicUnit=on
  Q-less QR Rotate First Element To Real1 : Subsystem  TreatAsAtomicUnit=on  mask(Rotate First Element To Real){n=n, pivot=pivot}
      mask prompts: n "fixed:emblib:ColumnsInA"
      mask help: fixed:emblib:RotateFirstElementToRealDescription
      mask DialogControl n Prompt: Number of columns in matrix A
  Set Element To Zero1 : Subsystem  mask(Set Element To Zero){n=n, pivot=pivot}
      mask prompts: n "fixed:emblib:ColumnsInA"
      mask help: fixed:emblib:SetElementToZeroDescription
      mask DialogControl n Prompt: Number of columns in matrix A
  Terminator3 : Terminator
  Unit Delay Enabled Synchronous1 : hdlsllib/Discrete/Unit Delay Enabled Synchronous  InitialCondition=0.0  SampleTime=-1
      settings: SourceProductBaseCode=SL
  Unit Delay Enabled Synchronous3 : hdlsllib/Discrete/Unit Delay Enabled Synchronous  InitialCondition=0.0  SampleTime=-1
      settings: SourceProductBaseCode=SL
  ValidIn to Ready Logic : Subsystem
  ValidIn to Ready Logic1 : Subsystem
  xOut : Outport  VectorParamsAs1DForOutWhenUnconnected=off
  yOut : Outport  Port=2  VectorParamsAs1DForOutWhenUnconnected=off
  validOut : Outport  Port=3  VectorParamsAs1DForOutWhenUnconnected=off
  ready : Outport  Port=4  VectorParamsAs1DForOutWhenUnconnected=off
  wires:
  Delay6/1 -> xOut/1
  Complex Partial-Systolic Q-less QR CORDIC Row Rotation/1(xOut) -> Delay17/1
  Q-less QR 2nd and 3rd Quadrant Compensation/1(xOut) -> Delay/1
  Q-less QR 2nd and 3rd Quadrant Compensation/2(yOut) -> Delay1/1
  Delay/1 -> Complex Partial-Systolic Q-less QR CORDIC Row Rotation/1(x)
  Q-less QR Rotate First Element To Real1/2(validOut) -> Unit Delay Enabled Synchronous3/2, Delay16/1
  Q-less QR Rotate First Element To Real1/1(xOut) -> Delay2/1
  Delay1/1 -> Complex Partial-Systolic Q-less QR CORDIC Row Rotation/2(y)
  restart/1 -> Q-less QR Rotate First Element To Real1/3(restart), Complex Partial-Systolic Q-less QR CORDIC Row Rotation/4(restart)
  Delay5/1 -> ValidIn to Ready Logic/2(validIn), Complex Partial-Systolic Q-less QR CORDIC Row Rotation/3(validIn)
  Complex Partial-Systolic Q-less QR CORDIC Row Rotation/4(ready) -> ValidIn to Ready Logic/1(readyIn)
  Complex Partial-Systolic Q-less QR CORDIC Row Rotation/3(validOut) -> Delay21/1
  Complex Partial-Systolic Q-less QR CORDIC Row Rotation/2(yOut) -> Delay18/1
  y/1 -> Delay3/1
  Delay10/1 -> validOut/1
  ValidIn to Ready Logic/1(readyOut) -> ValidIn to Ready Logic1/1(readyIn)
  Delay7/1 -> Set Element To Zero1/1(u)
  Q-less QR Rotate First Element To Real1/3(ready) -> Terminator3/1
  ValidIn to Ready Logic1/1(readyOut) -> ready/1
  Delay21/1 -> Delay10/1
  Delay18/1 -> Inverse CORDIC Gain1/1(u)
  Delay17/1 -> Inverse CORDIC Gain4/1(u)
  Inverse CORDIC Gain4/1(y) -> Delay6/1
  Inverse CORDIC Gain1/1(y) -> Delay7/1
  validIn/1 -> Unit Delay Enabled Synchronous1/2, Delay8/1
  Delay16/1 -> ValidIn to Ready Logic1/2(validIn), Delay5/1
  Delay2/1 -> Q-less QR 2nd and 3rd Quadrant Compensation/2(y)
  Unit Delay Enabled Synchronous3/1 -> Q-less QR 2nd and 3rd Quadrant Compensation/1(x)
  Unit Delay Enabled Synchronous1/1 -> Unit Delay Enabled Synchronous3/1
  x/1 -> Unit Delay Enabled Synchronous1/1
  Delay3/1 -> Q-less QR Rotate First Element To Real1/1(x)
  Delay8/1 -> Q-less QR Rotate First Element To Real1/2(validIn)
  Set Element To Zero1/1(y) -> yOut/1

== system qless_forgetting_factor_16x16/MVDR_QLess_HDL/Complex Partial-Systolic Matrix Solve Using Q-less QR Decomposition with Forgetting Factor Manually Tiled n=16/Complex Partial-Systolic Q-less QR with Forgetting Factor/Complex Partial-Systolic Q-less QR with Forgetting Factor Manually tiled/Complex Partial-Systolic Q-less QR Decomposition with Forgetting Factor Section Constant pivot11/Partial-Systolic Q-less QR with Forgetting Factor Memory Controller ==
  xIn : Inport
  aIn : Inport  Port=2
  validIn : Inport  Port=3
  validElim : Inport  Port=4
  restart : Inport  Port=5
  Delay{,2..4,6} (5 alike) : Delay  DelayLength=1
  MATLAB Function : MATLAB Function  TreatAsAtomicUnit=on
  xOut : Outport  VectorParamsAs1DForOutWhenUnconnected=off
  yOut : Outport  Port=2  VectorParamsAs1DForOutWhenUnconnected=off
  process : Outport  Port=3  VectorParamsAs1DForOutWhenUnconnected=off
  validOut : Outport  Port=4  VectorParamsAs1DForOutWhenUnconnected=off
  ready : Outport  Port=5  VectorParamsAs1DForOutWhenUnconnected=off
  wires:
  Delay/1 -> MATLAB Function/1(xIn)
  Delay2/1 -> MATLAB Function/2(aIn)
  Delay3/1 -> MATLAB Function/3(validIn)
  Delay4/1 -> MATLAB Function/4(validRowRotationInput)
  Delay6/1 -> MATLAB Function/5(restart)
  xIn/1 -> Delay/1  "A"
  aIn/1 -> Delay2/1
  validIn/1 -> Delay3/1  "validIn"
  validElim/1 -> Delay4/1  "validElim"
  restart/1 -> Delay6/1  "validElim"
  MATLAB Function/1(xOut) -> xOut/1
  MATLAB Function/2(yOut) -> yOut/1
  MATLAB Function/3(processRowRotations) -> process/1
  MATLAB Function/4(validOut) -> validOut/1
  MATLAB Function/5(ready) -> ready/1

== system qless_forgetting_factor_16x16/MVDR_QLess_HDL/Complex Partial-Systolic Matrix Solve Using Q-less QR Decomposition with Forgetting Factor Manually Tiled n=16/Complex Partial-Systolic Q-less QR with Forgetting Factor/Complex Partial-Systolic Q-less QR with Forgetting Factor Manually tiled/Complex Partial-Systolic Q-less QR Decomposition with Forgetting Factor Section Constant pivot11/Same Datatype ==
  Data : Inport
  Reference : Inport  Port=2
  Data Type Duplicate : DataTypeDuplicate
  DataOut : Outport  VectorParamsAs1DForOutWhenUnconnected=off
  wires:
  Reference/1 -> Data Type Duplicate/2
  Data/1 -> DataOut/1, Data Type Duplicate/1
